simulink model "order1_math_model"  (R2021a)
settings: Solver=FixedStepAuto  StartTime=0.0  StopTime=10  FixedStep=1e-4  RelTol=1e-4
values from neighbouring files (symbols this model uses):
  g = 9.8    [order1_all_observer_sfun.m]    (also in order1_calc.m; order1_min_observer_sfun.m)
  I = 1/3*m*l^2    (= 0.00833333333333)    [order1_all_observer_sfun.m]    (also in order1_calc.m; order1_min_observer_sfun.m)
  K = [-1.1020, -2.2041, -37.5147, -8.2194]    [order1_all_observer_sfun.m]    (also in order1_calc.m = K2)
  K_lqr = lqr(A,B,Q,R)    [order1_calc.m]
  l = 0.5    [order1_all_observer_sfun.m]    (also in order1_calc.m; order1_min_observer_sfun.m)
  m = 0.1    [order1_all_observer_sfun.m]    (also in order1_calc.m; order1_min_observer_sfun.m)
  M = 2    [order1_all_observer_sfun.m]    (also in order1_calc.m; order1_min_observer_sfun.m)
settings Model: Creator=cc  LastModifiedBy=cc

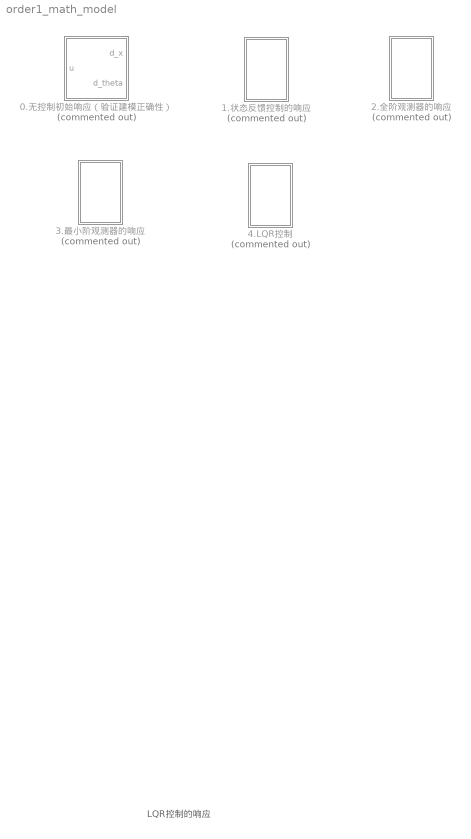
== system order1_math_model ==
  note: LQR控制的响应
  0.无控制初始响应（验证建模正确性） : Subsystem  Commented=on
  1.状态反馈控制的响应 : Subsystem  Commented=on
  2.全阶观测器的响应 : Subsystem  Commented=on
  3.最小阶观测器的响应 : Subsystem  Commented=on
  4.LQR控制 : Subsystem  Commented=on

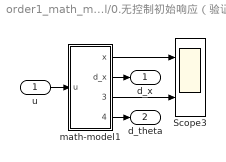
== system order1_math_model/0.无控制初始响应（验证建模正确性） ==
  u : Inport
  Scope3 : Scope  NumInputPorts=2
  math-model1 : Subsystem  mask{theta_0=30/180*pi, x_0=0}
  d_x : Outport
  d_theta : Outport  Port=2
  wires:
  math-model1/2(d_x) -> d_x/1
  math-model1/1(x) -> Scope3/1
  math-model1/3(theta) -> Scope3/2
  math-model1/4(d_theta) -> d_theta/1
  u/1 -> math-model1/1(u)

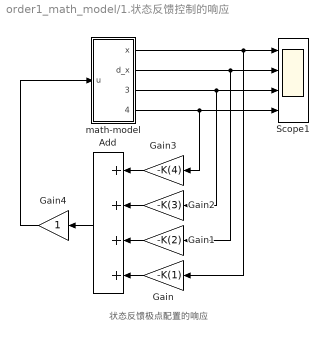
== system order1_math_model/1.状态反馈控制的响应 ==
  note: 状态反馈极点配置的响应
  Add : Sum  Inputs=++++
  Gain : Gain  Gain=-K(1)
  Gain1 : Gain  Gain=-K(2)
  Gain2 : Gain  Gain=-K(3)
  Gain3 : Gain  Gain=-K(4)
  Gain4 : Gain
  Scope1 : Scope  NumInputPorts=4
  math-model : Subsystem  mask{theta_0=5/180*pi, x_0=0}
  wires:
  math-model/2(d_x) -> Gain1/1, Scope1/2
  math-model/3(theta) -> Scope1/3, Gain2/1
  math-model/1(x) -> Gain/1, Scope1/1
  Gain3/1 -> Add/1
  Gain2/1 -> Add/2
  Gain4/1 -> math-model/1(u)
  math-model/4(d_theta) -> Scope1/4, Gain3/1
  Gain/1 -> Add/4
  Gain1/1 -> Add/3
  Add/1 -> Gain4/1

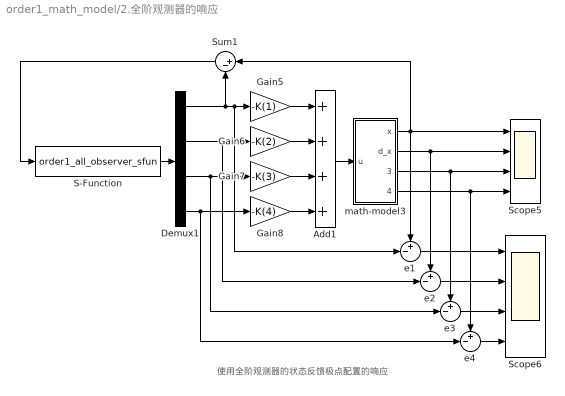
== system order1_math_model/2.全阶观测器的响应 ==
  note: 使用全阶观测器的状态反馈极点配置的响应
  Add1 : Sum  Inputs=++++
  Demux1 : Demux
  Gain5 : Gain  Gain=-K(1)
  Gain6 : Gain  Gain=-K(2)
  Gain7 : Gain  Gain=-K(3)
  Gain8 : Gain  Gain=-K(4)
  S-Function : S-Function  FunctionName=order1_all_observer_sfun  Parameters=0; 0  SFunctionDeploymentMode=off  EnableBusSupport=off
  Scope5 : Scope  NumInputPorts=4
  Scope6 : Scope  NumInputPorts=4
  Sum1 : Sum  Inputs=|+-
  e{1..4} (4 alike) : Sum  Inputs=+-|
  math-model3 : Subsystem  mask{theta_0=5/180*pi, x_0=0}
  wires:
  Add1/1 -> math-model3/1(u)
  Demux1/1 -> Gain5/1, e1/2, Sum1/2
  Gain7/1 -> Add1/3
  math-model3/2(d_x) -> Scope5/2, e2/1
  e3/1 -> Scope6/3
  math-model3/3(theta) -> Scope5/3, e3/1
  math-model3/1(x) -> Scope5/1, e1/1, Sum1/1
  e2/1 -> Scope6/2
  e4/1 -> Scope6/4
  Demux1/2 -> e2/2, Gain6/1
  Demux1/4 -> e4/2, Gain8/1
  Gain5/1 -> Add1/1
  e1/1 -> Scope6/1
  Demux1/3 -> e3/2, Gain7/1
  Gain8/1 -> Add1/4
  math-model3/4(d_theta) -> Scope5/4, e4/1
  S-Function/1 -> Demux1/1
  Sum1/1 -> S-Function/1
  Gain6/1 -> Add1/2

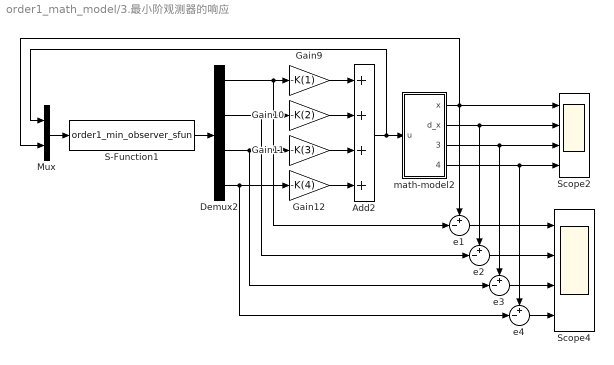
== system order1_math_model/3.最小阶观测器的响应 ==
  Add2 : Sum  Inputs=++++
  Demux2 : Demux
  Gain10 : Gain  Gain=-K(2)
  Gain11 : Gain  Gain=-K(3)
  Gain12 : Gain  Gain=-K(4)
  Gain9 : Gain  Gain=-K(1)
  Mux : Mux  Inputs=2
  S-Function1 : S-Function  FunctionName=order1_min_observer_sfun  Parameters=0; 0  SFunctionDeploymentMode=off  EnableBusSupport=off
  Scope2 : Scope  NumInputPorts=4
  Scope4 : Scope  NumInputPorts=4
  e{1..4} (4 alike) : Sum  Inputs=+-|
  math-model2 : Subsystem  mask{theta_0=5/180*pi, x_0=0}
  wires:
  Demux2/4 -> e4/2, Gain12/1
  Mux/1 -> S-Function1/1
  Add2/1 -> Mux/1, math-model2/1(u)
  e4/1 -> Scope4/4
  math-model2/1(x) -> e1/1, Mux/2, Scope2/1
  Demux2/1 -> Gain9/1, e1/2
  S-Function1/1 -> Demux2/1
  Demux2/3 -> e3/2, Gain11/1
  math-model2/4(d_theta) -> Scope2/4, e4/1
  e3/1 -> Scope4/3
  e1/1 -> Scope4/1
  math-model2/3(theta) -> Scope2/3, e3/1
  math-model2/2(d_x) -> Scope2/2, e2/1
  Gain10/1 -> Add2/2
  Demux2/2 -> e2/2, Gain10/1
  Gain11/1 -> Add2/3
  Gain12/1 -> Add2/4
  Gain9/1 -> Add2/1
  e2/1 -> Scope4/2

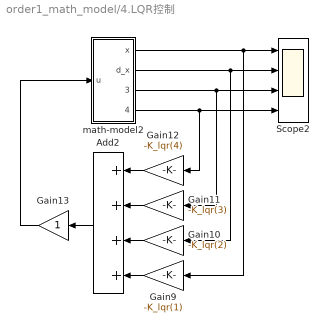
== system order1_math_model/4.LQR控制 ==
  Add2 : Sum  Inputs=++++
  Gain10 : Gain  Gain=-K_lqr(2)
  Gain11 : Gain  Gain=-K_lqr(3)
  Gain12 : Gain  Gain=-K_lqr(4)
  Gain13 : Gain
  Gain9 : Gain  Gain=-K_lqr(1)
  Scope2 : Scope  NumInputPorts=4
  math-model2 : Subsystem  mask{theta_0=5/180*pi, x_0=0}
  wires:
  Gain13/1 -> math-model2/1(u)
  math-model2/2(d_x) -> Gain10/1, Scope2/2
  Gain9/1 -> Add2/4
  math-model2/3(theta) -> Scope2/3, Gain11/1
  math-model2/4(d_theta) -> Scope2/4, Gain12/1
  Add2/1 -> Gain13/1
  Gain11/1 -> Add2/2
  Gain12/1 -> Add2/1
  math-model2/1(x) -> Gain9/1, Scope2/1
  Gain10/1 -> Add2/3

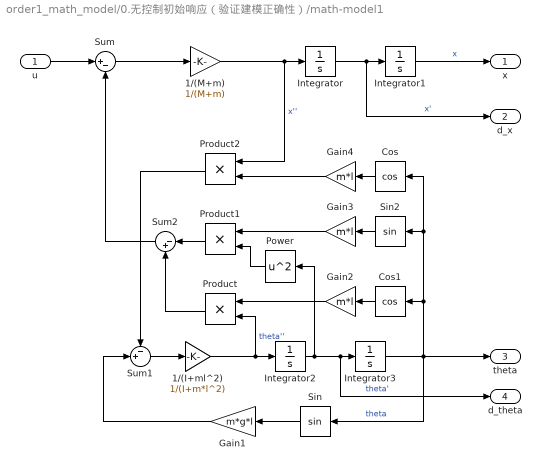
== system order1_math_model/0.无控制初始响应（验证建模正确性）/math-model1 ==
  u : Inport
  1/(I+ml^2) : Gain  Gain=1/(I+m*l^2)
  1/(M+m) : Gain  Gain=1/(M+m)
  Cos : Trigonometry  Operator=cos
  Cos1 : Trigonometry  Operator=cos
  Gain1 : Gain  Gain=m*g*l
  Gain2 : Gain  Gain=m*l
  Gain3 : Gain  Gain=m*l
  Gain4 : Gain  Gain=m*l
  Integrator : Integrator
  Integrator1 : Integrator  InitialCondition=x_0
  Integrator2 : Integrator
  Integrator3 : Integrator  InitialCondition=theta_0
  Power : Math  Operator=square  SaturateOnIntegerOverflow=on
  Product : Product
  Product1 : Product
  Product2 : Product
  Sin : Trigonometry
  Sin2 : Trigonometry
  Sum : Sum  Inputs=|+-
  Sum1 : Sum  Inputs=-+|
  Sum2 : Sum  Inputs=|-+
  x : Outport  VectorParamsAs1DForOutWhenUnconnected=off
  d_x : Outport  Port=2  VectorParamsAs1DForOutWhenUnconnected=off
  theta : Outport  Port=3  VectorParamsAs1DForOutWhenUnconnected=off
  d_theta : Outport  Port=4  VectorParamsAs1DForOutWhenUnconnected=off
  wires:
  Sum/1 -> 1/(M+m)/1
  Product2/1 -> Sum1/1
  Cos1/1 -> Gain2/1
  Product1/1 -> Sum2/1
  1/(M+m)/1 -> Product2/1, Integrator/1  "x''"
  Sin/1 -> Gain1/1
  u/1 -> Sum/1
  Gain2/1 -> Product/1
  1/(I+ml^2)/1 -> Product/2, Integrator2/1  "theta''"
  Integrator3/1 -> theta/1, Cos/1, Sin2/1, Cos1/1, Sin/1  "theta"
  Integrator2/1 -> d_theta/1, Integrator3/1, Power/1  "theta'"
  Gain1/1 -> Sum1/2
  Integrator/1 -> d_x/1, Integrator1/1  "x'"
  Gain4/1 -> Product2/2
  Gain3/1 -> Product1/1
  Power/1 -> Product1/2
  Sum1/1 -> 1/(I+ml^2)/1
  Integrator1/1 -> x/1  "x"
  Sum2/1 -> Sum/2
  Product/1 -> Sum2/2
  Cos/1 -> Gain4/1
  Sin2/1 -> Gain3/1

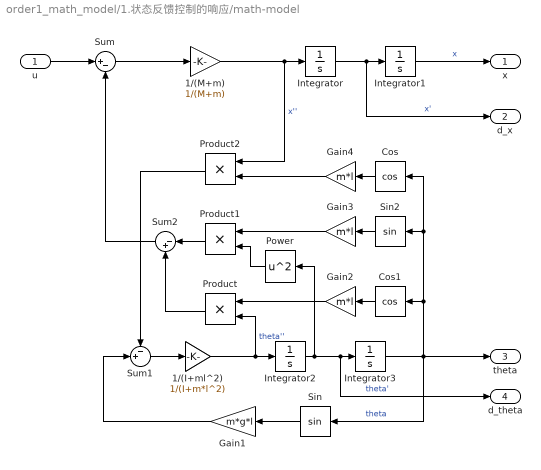
== system order1_math_model/1.状态反馈控制的响应/math-model ==
  u : Inport
  1/(I+ml^2) : Gain  Gain=1/(I+m*l^2)
  1/(M+m) : Gain  Gain=1/(M+m)
  Cos : Trigonometry  Operator=cos
  Cos1 : Trigonometry  Operator=cos
  Gain1 : Gain  Gain=m*g*l
  Gain2 : Gain  Gain=m*l
  Gain3 : Gain  Gain=m*l
  Gain4 : Gain  Gain=m*l
  Integrator : Integrator
  Integrator1 : Integrator  InitialCondition=x_0
  Integrator2 : Integrator
  Integrator3 : Integrator  InitialCondition=theta_0
  Power : Math  Operator=square  SaturateOnIntegerOverflow=on
  Product : Product
  Product1 : Product
  Product2 : Product
  Sin : Trigonometry
  Sin2 : Trigonometry
  Sum : Sum  Inputs=|+-
  Sum1 : Sum  Inputs=-+|
  Sum2 : Sum  Inputs=|-+
  x : Outport  VectorParamsAs1DForOutWhenUnconnected=off
  d_x : Outport  Port=2  VectorParamsAs1DForOutWhenUnconnected=off
  theta : Outport  Port=3  VectorParamsAs1DForOutWhenUnconnected=off
  d_theta : Outport  Port=4  VectorParamsAs1DForOutWhenUnconnected=off
  wires:
  Sum/1 -> 1/(M+m)/1
  Product2/1 -> Sum1/1
  Cos1/1 -> Gain2/1
  Product1/1 -> Sum2/1
  1/(M+m)/1 -> Product2/1, Integrator/1  "x''"
  Sin/1 -> Gain1/1
  u/1 -> Sum/1
  Gain2/1 -> Product/1
  1/(I+ml^2)/1 -> Product/2, Integrator2/1  "theta''"
  Integrator3/1 -> theta/1, Cos/1, Sin2/1, Cos1/1, Sin/1  "theta"
  Integrator2/1 -> d_theta/1, Integrator3/1, Power/1  "theta'"
  Gain1/1 -> Sum1/2
  Integrator/1 -> d_x/1, Integrator1/1  "x'"
  Gain4/1 -> Product2/2
  Gain3/1 -> Product1/1
  Power/1 -> Product1/2
  Sum1/1 -> 1/(I+ml^2)/1
  Integrator1/1 -> x/1  "x"
  Sum2/1 -> Sum/2
  Product/1 -> Sum2/2
  Cos/1 -> Gain4/1
  Sin2/1 -> Gain3/1

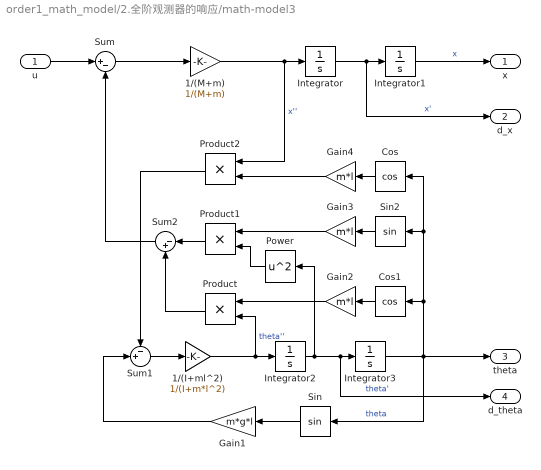
== system order1_math_model/2.全阶观测器的响应/math-model3 ==
  u : Inport
  1/(I+ml^2) : Gain  Gain=1/(I+m*l^2)
  1/(M+m) : Gain  Gain=1/(M+m)
  Cos : Trigonometry  Operator=cos
  Cos1 : Trigonometry  Operator=cos
  Gain1 : Gain  Gain=m*g*l
  Gain2 : Gain  Gain=m*l
  Gain3 : Gain  Gain=m*l
  Gain4 : Gain  Gain=m*l
  Integrator : Integrator
  Integrator1 : Integrator  InitialCondition=x_0
  Integrator2 : Integrator
  Integrator3 : Integrator  InitialCondition=theta_0
  Power : Math  Operator=square  SaturateOnIntegerOverflow=on
  Product : Product
  Product1 : Product
  Product2 : Product
  Sin : Trigonometry
  Sin2 : Trigonometry
  Sum : Sum  Inputs=|+-
  Sum1 : Sum  Inputs=-+|
  Sum2 : Sum  Inputs=|-+
  x : Outport  VectorParamsAs1DForOutWhenUnconnected=off
  d_x : Outport  Port=2  VectorParamsAs1DForOutWhenUnconnected=off
  theta : Outport  Port=3  VectorParamsAs1DForOutWhenUnconnected=off
  d_theta : Outport  Port=4  VectorParamsAs1DForOutWhenUnconnected=off
  wires:
  Sum/1 -> 1/(M+m)/1
  Product2/1 -> Sum1/1
  Cos1/1 -> Gain2/1
  Product1/1 -> Sum2/1
  1/(M+m)/1 -> Product2/1, Integrator/1  "x''"
  Sin/1 -> Gain1/1
  u/1 -> Sum/1
  Gain2/1 -> Product/1
  1/(I+ml^2)/1 -> Product/2, Integrator2/1  "theta''"
  Integrator3/1 -> theta/1, Cos/1, Sin2/1, Cos1/1, Sin/1  "theta"
  Integrator2/1 -> d_theta/1, Integrator3/1, Power/1  "theta'"
  Gain1/1 -> Sum1/2
  Integrator/1 -> d_x/1, Integrator1/1  "x'"
  Gain4/1 -> Product2/2
  Gain3/1 -> Product1/1
  Power/1 -> Product1/2
  Sum1/1 -> 1/(I+ml^2)/1
  Integrator1/1 -> x/1  "x"
  Sum2/1 -> Sum/2
  Product/1 -> Sum2/2
  Cos/1 -> Gain4/1
  Sin2/1 -> Gain3/1

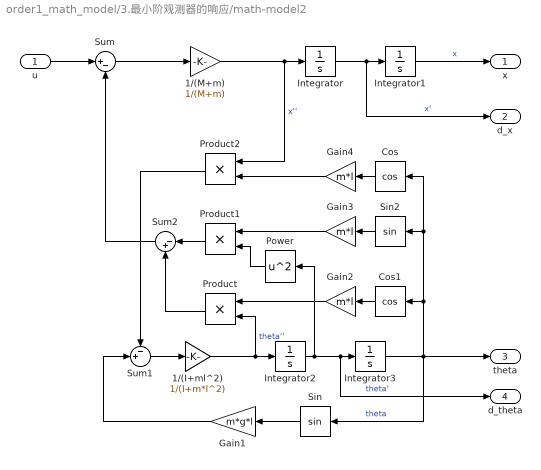
== system order1_math_model/3.最小阶观测器的响应/math-model2 ==
  u : Inport
  1/(I+ml^2) : Gain  Gain=1/(I+m*l^2)
  1/(M+m) : Gain  Gain=1/(M+m)
  Cos : Trigonometry  Operator=cos
  Cos1 : Trigonometry  Operator=cos
  Gain1 : Gain  Gain=m*g*l
  Gain2 : Gain  Gain=m*l
  Gain3 : Gain  Gain=m*l
  Gain4 : Gain  Gain=m*l
  Integrator : Integrator
  Integrator1 : Integrator  InitialCondition=x_0
  Integrator2 : Integrator
  Integrator3 : Integrator  InitialCondition=theta_0
  Power : Math  Operator=square  SaturateOnIntegerOverflow=on
  Product : Product
  Product1 : Product
  Product2 : Product
  Sin : Trigonometry
  Sin2 : Trigonometry
  Sum : Sum  Inputs=|+-
  Sum1 : Sum  Inputs=-+|
  Sum2 : Sum  Inputs=|-+
  x : Outport  VectorParamsAs1DForOutWhenUnconnected=off
  d_x : Outport  Port=2  VectorParamsAs1DForOutWhenUnconnected=off
  theta : Outport  Port=3  VectorParamsAs1DForOutWhenUnconnected=off
  d_theta : Outport  Port=4  VectorParamsAs1DForOutWhenUnconnected=off
  wires:
  Sum/1 -> 1/(M+m)/1
  Product2/1 -> Sum1/1
  Cos1/1 -> Gain2/1
  Product1/1 -> Sum2/1
  1/(M+m)/1 -> Product2/1, Integrator/1  "x''"
  Sin/1 -> Gain1/1
  u/1 -> Sum/1
  Gain2/1 -> Product/1
  1/(I+ml^2)/1 -> Product/2, Integrator2/1  "theta''"
  Integrator3/1 -> theta/1, Cos/1, Sin2/1, Cos1/1, Sin/1  "theta"
  Integrator2/1 -> d_theta/1, Integrator3/1, Power/1  "theta'"
  Gain1/1 -> Sum1/2
  Integrator/1 -> d_x/1, Integrator1/1  "x'"
  Gain4/1 -> Product2/2
  Gain3/1 -> Product1/1
  Power/1 -> Product1/2
  Sum1/1 -> 1/(I+ml^2)/1
  Integrator1/1 -> x/1  "x"
  Sum2/1 -> Sum/2
  Product/1 -> Sum2/2
  Cos/1 -> Gain4/1
  Sin2/1 -> Gain3/1

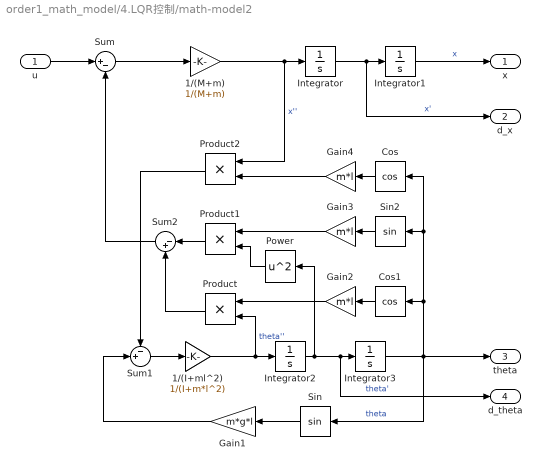
== system order1_math_model/4.LQR控制/math-model2 ==
  u : Inport
  1/(I+ml^2) : Gain  Gain=1/(I+m*l^2)
  1/(M+m) : Gain  Gain=1/(M+m)
  Cos : Trigonometry  Operator=cos
  Cos1 : Trigonometry  Operator=cos
  Gain1 : Gain  Gain=m*g*l
  Gain2 : Gain  Gain=m*l
  Gain3 : Gain  Gain=m*l
  Gain4 : Gain  Gain=m*l
  Integrator : Integrator
  Integrator1 : Integrator  InitialCondition=x_0
  Integrator2 : Integrator
  Integrator3 : Integrator  InitialCondition=theta_0
  Power : Math  Operator=square  SaturateOnIntegerOverflow=on
  Product : Product
  Product1 : Product
  Product2 : Product
  Sin : Trigonometry
  Sin2 : Trigonometry
  Sum : Sum  Inputs=|+-
  Sum1 : Sum  Inputs=-+|
  Sum2 : Sum  Inputs=|-+
  x : Outport  VectorParamsAs1DForOutWhenUnconnected=off
  d_x : Outport  Port=2  VectorParamsAs1DForOutWhenUnconnected=off
  theta : Outport  Port=3  VectorParamsAs1DForOutWhenUnconnected=off
  d_theta : Outport  Port=4  VectorParamsAs1DForOutWhenUnconnected=off
  wires:
  Sum/1 -> 1/(M+m)/1
  Product2/1 -> Sum1/1
  Cos1/1 -> Gain2/1
  Product1/1 -> Sum2/1
  1/(M+m)/1 -> Product2/1, Integrator/1  "x''"
  Sin/1 -> Gain1/1
  u/1 -> Sum/1
  Gain2/1 -> Product/1
  1/(I+ml^2)/1 -> Product/2, Integrator2/1  "theta''"
  Integrator3/1 -> theta/1, Cos/1, Sin2/1, Cos1/1, Sin/1  "theta"
  Integrator2/1 -> d_theta/1, Integrator3/1, Power/1  "theta'"
  Gain1/1 -> Sum1/2
  Integrator/1 -> d_x/1, Integrator1/1  "x'"
  Gain4/1 -> Product2/2
  Gain3/1 -> Product1/1
  Power/1 -> Product1/2
  Sum1/1 -> 1/(I+ml^2)/1
  Integrator1/1 -> x/1  "x"
  Sum2/1 -> Sum/2
  Product/1 -> Sum2/2
  Cos/1 -> Gain4/1
  Sin2/1 -> Gain3/1
